simulink model "PV_Array_Code_Gen_PIL"  (R2023b)
settings: Solver=FixedStepAuto  StartTime=0.0  StopTime=86400  FixedStep=1  RelTol=1e-3  EnableMultiTasking=on
libraries: spsSeriesRLCBranchLib x5, spsIdealSwitchLib x3, stm32blockslib x2, spsCurrentMeasurementLib x1, spsDiodeLib x1, spsMosfetLib x1, spsPVArrayLib x1, eePwmGenerator x1, spsVoltageMeasurementLib x1, sps_lib x1
settings Model: STM32="{\"UARTWrite\":{\"ID\":\"PV_Array_Code_Gen:122\"},\"UARTRead\":{\"ID\":\"PV_Array_Code_Gen:121\"}}"  SimulationMode=external  Creator=chate  LastModifiedBy=chate
settings OptimizationCC: EnhancedBackFolding=on  PassReuseOutputArgsAs=Individual arguments  ZeroExternalMemoryAtStartup=off  ZeroInternalMemoryAtStartup=off  MaxStackSize=64  OptimizeBlockOrder=speed  DifferentSizesBufferReuse=on  OptimizationCustomize=off  EfficientTunableParamExpr=on
settings DebuggingCC: AlgebraicLoopMsg=none  ParameterTunabilityLossMsg=error
settings HardwareCC: ProdBitPerPointer=32  ProdBitPerSizeT=32  ProdBitPerPtrDiffT=32  ProdLargestAtomicInteger=Long  ProdLargestAtomicFloat=Double  ProdWordSize=32  ProdLongLongMode=on  ProdHWDeviceType=ARM Compatible->ARM Cortex
settings SFSimCC: MATLABDynamicMemAlloc=off
settings RTWCC: Description=Embedded Coder  SystemTargetFile=ert.tlc  HardwareBoard=STM32F4xx Based  TemplateMakefile=ert_default_tmf  Toolchain=GNU Tools for ARM Embedded Processors  CreateSILPILBlock=PIL
settings CodeAppCC: ForceParamTrailComments=on  IgnoreCustomStorageClasses=off  OperatorAnnotations=on  SimulinkDataObjDesc=on  SFDataObjDesc=on  InsertBlockDesc=on
settings ERTTargetCC: CodeReplacementLibrary=ARM Cortex-M  SupportContinuousTime=on  ExtModeTransport=3  ExtModeStaticAlloc=on  ExtModeStaticAllocSize=2048  ExtModeMexFile=ext_xcp  ExtModeIntrfLevel=Level2 - Open

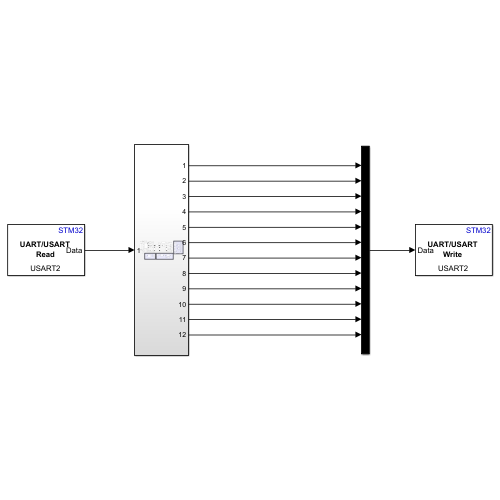
[thumbnail: Simulink's stored preview of the top-level diagram]
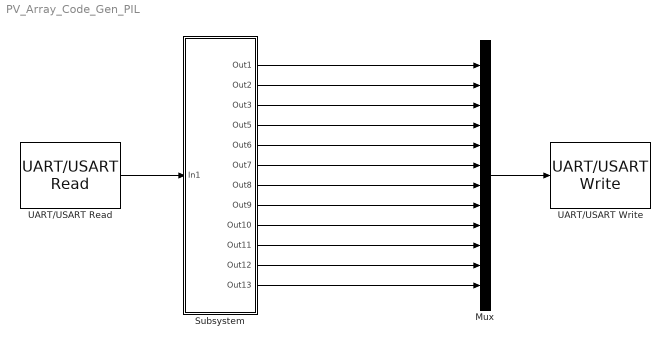
== system PV_Array_Code_Gen_PIL ==
  Mux : Mux  Inputs=12
  Subsystem : Subsystem
  UART/USART Read : stm32blockslib/UART//USART Read  Priority=0  UARTModule=USART2  DataType=double  DataLength=2  BlockingMode=off  BlockingTimeout=0.1  OutputLength=off  OutputStatus=off  SampleTime=1
      settings: LibrarySourceBlock=stm32f4xxblockslib/UART//USART Read
  UART/USART Write : stm32blockslib/UART//USART Write  Priority=1  UARTModule=USART2  LengthOfDataToSend=off  BlockingMode=off  BlockingTimeout=0.1  OutputStatus=off
      settings: LibrarySourceBlock=stm32f4xxblockslib/UART//USART Write
  wires:
  Subsystem/1(Out1) -> Mux/1
  Subsystem/2(Out2) -> Mux/2
  Subsystem/3(Out3) -> Mux/3
  Subsystem/4(Out5) -> Mux/4
  Subsystem/5(Out6) -> Mux/5
  Subsystem/6(Out7) -> Mux/6
  Subsystem/7(Out8) -> Mux/7
  Subsystem/8(Out9) -> Mux/8
  Subsystem/9(Out10) -> Mux/9
  Subsystem/10(Out11) -> Mux/10
  Subsystem/11(Out12) -> Mux/11
  Subsystem/12(Out13) -> Mux/12
  UART/USART Read/1 -> Subsystem/1(In1)
  Mux/1 -> UART/USART Write/1

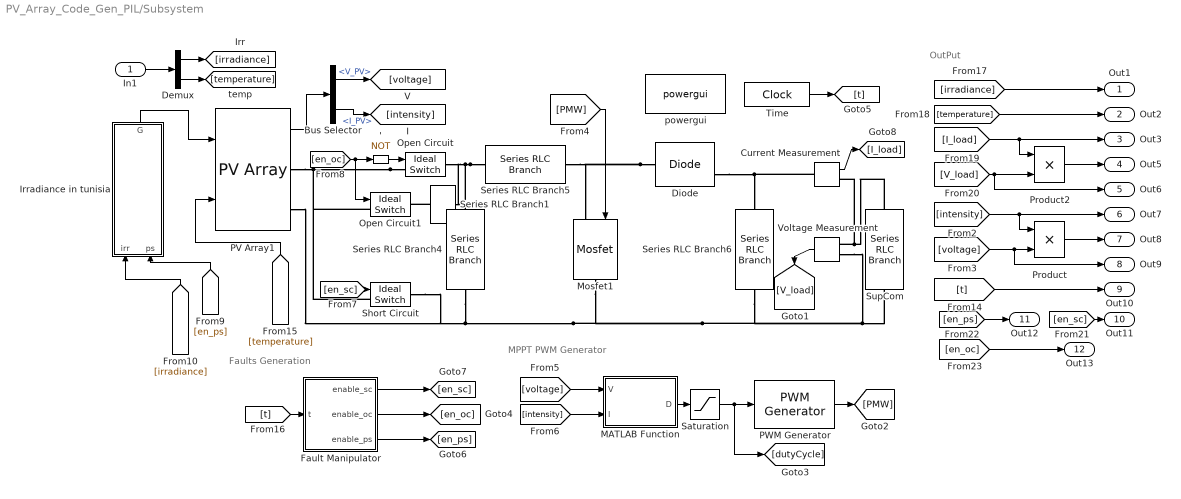
== system PV_Array_Code_Gen_PIL/Subsystem ==
  note: OutPut
  note: Faults Generation
  note: MPPT PWM Generator
  In1 : Inport
  ' : Logic  Operator=NOT  IconShape=distinctive  AllPortsSameDT=off  OutDataTypeStr=boolean
  Bus Selector : BusSelector  OutputSignals=V_PV,I_PV
  Current Measurement : spsCurrentMeasurementLib/Current Measurement  PhasorSimulation=off  OutputType=Complex  PSBequivalent=0
  Demux : Demux  Outputs=2
  Diode : spsDiodeLib/Diode  Ron=0.001  Lon=0  Vf=0.8  IC=0  UseSnubber=0  Rs=100  Cs=1e-7  Measurements=on
  Fault Manipulator : MATLAB Function  TreatAsAtomicUnit=on
  Irradiance in tunisia : MATLAB Function  TreatAsAtomicUnit=on
  MATLAB Function : MATLAB Function  TreatAsAtomicUnit=on
  Mosfet1 : spsMosfetLib/Mosfet  Ron=1e-3  Lon=0  Rd=1e-3  Vfd=0  IC=0  Rs=100  Cs=1e-7  Measurements=off
  Open Circuit : spsIdealSwitchLib/Ideal Switch  Ron=0.000001  Lon=0  IC=1  Rs=0  Cs=0  Measurements=off
  Open Circuit1 : spsIdealSwitchLib/Ideal Switch  Ron=0.000001  Lon=0  IC=0  Rs=0  Cs=0  Measurements=off
  PV Array1 : spsPVArrayLib/PV Array  Npar=3  Nser=15  PlotType=array @ 1000 W/m2 & specified temperatures  S_vec="[ 1000  500  100 ]"  Temp_C_vec="[ 45 25  ]"  ModuleName=User-defined  PlotWhenSelected=off  Pm=451.278  Ncell=60  Voc=49.8  Isc=11.56  Vm=41.1  Im=10.98  beta_Voc_pc=-0.36099  alpha_Isc_pc=0.102  beta_Voc=-0.17977  alpha_Isc=0.011791  IL=11.6189  I0=4.2897e-10  nI=1.3452  Rsh=602.3017  Rs=0.22981  RobustModel=off  RobustCellTemperature=25  BAL=on  Tc=1e-6  Tfilter=5e-5
  PWM Generator : eePwmGenerator/PWM Generator  CarrCount=Up  Tper=10  Tdelay=0  Ts=1
  Product : Product
  Product2 : Product
  Saturation : Saturate  UpperLimit=1  LowerLimit=0
  Series RLC Branch1 : spsSeriesRLCBranchLib/Series RLC Branch  LConnTagsString=__new0  RConnTagsString=__new0  BranchType=R  Resistance=7.3  Inductance=1.63e-2  SetiL0=off  InitialCurrent=0  Capacitance=1e-3  Setx0=off  InitialVoltage=0  Measurements=None
  Series RLC Branch4 : spsSeriesRLCBranchLib/Series RLC Branch  LConnTagsString=__new0  RConnTagsString=__new0  BranchType=C  Resistance=1  Inductance=1e-3  SetiL0=off  InitialCurrent=0  Capacitance=46.6e-2  Setx0=off  InitialVoltage=0  Measurements=None
  Series RLC Branch5 : spsSeriesRLCBranchLib/Series RLC Branch  LConnTagsString=__new0  RConnTagsString=__new0  BranchType=L  Resistance=1  Inductance=1.63e-2  SetiL0=off  InitialCurrent=0  Capacitance=1e-3  Setx0=off  InitialVoltage=0  Measurements=None
  Series RLC Branch6 : spsSeriesRLCBranchLib/Series RLC Branch  LConnTagsString=__new0  RConnTagsString=__new0  BranchType=C  Resistance=1  Inductance=1e-3  SetiL0=off  InitialCurrent=0  Capacitance=63e-2  Setx0=off  InitialVoltage=0  Measurements=None
  Short Circuit : spsIdealSwitchLib/Ideal Switch  Ron=0.000001  Lon=0  IC=0  Rs=0  Cs=0  Measurements=off
  SupCom : spsSeriesRLCBranchLib/Series RLC Branch  LConnTagsString=__new0  RConnTagsString=__new0  BranchType=R  Resistance=18.5  Inductance=1e-3  SetiL0=off  InitialCurrent=0  Capacitance=1e-3  Setx0=off  InitialVoltage=0  Measurements=None
  Time : DigitalClock
  Voltage Measurement : spsVoltageMeasurementLib/Voltage Measurement  PhasorSimulation=off  OutputType=Complex  PSBequivalent=0
  powergui : sps_lib/powergui  Priority=1  SimulationMode=Discrete  SampleTime=1  frequency=60  Iterations=50  frequencyindice=0  Pbase=100e6  ErrMax=1e-4  UnitsV=kV  UnitsW=MW  buscounter=0  FunctionMessages=off  echomessages=off  EnableUseOfTLC=off  CurrentSourceSwitches=off  DisableSnubberDevices=off  DisableRonSwitches=off  DisableVfSwitches=off  DisplayEquations=off  AutomaticDiscreteSolvers=off  SolverType=Tustin/Backward Euler (TBE)  Interpol=off  ExternalGateDelay=off  methode=off  Ts=100  x0status=blocks  SPID=on  SwTol=0  HookPort=off  NonlinearTolerance=1e-4  nMaxIteration=100  ContinueOnMaxIteration=off  RestoreLinks=warning  ResistiveCurrentMeasurement=off  Frange=[0:2:500]  Ylog=off  Xlog=on  ShowGrid=off  save=off  variable=ZData  structure=0  ZoomFFT=off  StartTime=0.0  cycles=1  DisplayStyle=1  fundamental=60  FreqAxis=off  MaxFrequency=1000  frequencyindicesteady=1  RmsSteady=1  display=off
  Out1 : Outport
  Out2 : Outport  Port=2
  Out3 : Outport  Port=3
  Out5 : Outport  Port=4
  Out6 : Outport  Port=5
  Out7 : Outport  Port=6
  Out8 : Outport  Port=7
  Out9 : Outport  Port=8
  Out10 : Outport  Port=9
  Out11 : Outport  Port=10
  Out12 : Outport  Port=11
  Out13 : Outport  Port=12
  wires:
  [temperature] -> PV Array1/2
  [en_oc] -> '/1, Open Circuit1/1
  [intensity] -> MATLAB Function/2(I)
  [en_oc] -> Out13/1
  Fault Manipulator/3(enable_ps) -> [en_ps]
  Bus Selector/2 -> [intensity]  "<I_PV>"
  Fault Manipulator/2(enable_oc) -> [en_oc]
  Irradiance in tunisia/1(G) -> PV Array1/1
  [V_load] -> Out6/1, Product2/2
  Current Measurement/1 -> [I_load]
  [temperature] -> Out2/1
  Product/1 -> Out8/1
  Demux/1 -> [irradiance]
  [voltage] -> MATLAB Function/1(V)
  [I_load] -> Out3/1, Product2/1
  Voltage Measurement/1 -> [V_load]
  PWM Generator/1 -> [PMW]
  [PMW] -> Mosfet1/1
  MATLAB Function/1(D) -> Saturation/1
  Fault Manipulator/1(enable_sc) -> [en_sc]
  [voltage] -> Out9/1, Product/2
  [en_ps] -> Irradiance in tunisia/2(ps)
  PV Array1/1 -> Bus Selector/1
  [intensity] -> Out7/1, Product/1
  Bus Selector/1 -> [voltage]  "<V_PV>"
  Time/1 -> [t]
  [t] -> Fault Manipulator/1(t)
  [irradiance] -> Irradiance in tunisia/1(irr)
  Demux/2 -> [temperature]
  Saturation/1 -> PWM Generator/1, [dutyCycle]
  '/1 -> Open Circuit/1
  [en_sc] -> Out11/1
  [irradiance] -> Out1/1
  [en_sc] -> Short Circuit/1
  Product2/1 -> Out5/1
  In1/1 -> Demux/1
  [t] -> Out10/1
  [en_ps] -> Out12/1
  connections:
  Series RLC Branch5/LConn1 -- Series RLC Branch4/LConn1 -- Series RLC Branch1/RConn1 -- Open Circuit/RConn1
  Diode/RConn1 -- Current Measurement/LConn1 -- Series RLC Branch6/LConn1
  Open Circuit/LConn1 -- PV Array1/RConn1 -- Open Circuit1/LConn1 -- Short Circuit/LConn1
  Voltage Measurement/LConn1 -- SupCom/LConn1 -- Current Measurement/RConn1
  Diode/LConn1 -- Series RLC Branch5/RConn1 -- Mosfet1/LConn1
  Voltage Measurement/LConn2 -- Series RLC Branch6/RConn1 -- Mosfet1/RConn1 -- Series RLC Branch4/RConn1 -- Short Circuit/RConn1 -- PV Array1/RConn2 -- SupCom/RConn1
  Series RLC Branch1/LConn1 -- Open Circuit1/RConn1

== matlab function PV_Array_Code_Gen_PIL/Subsystem/Irradiance in tunisia ==
  data: irr input; G output; ps input
function G = irradiance_profile_tunisia(irr, ps)
    
    G = max(0, irr);

    if ps == 1
        G = 0.85 * G;  % Reduce irradiance to 85%
    end
end

== matlab function PV_Array_Code_Gen_PIL/Subsystem/Fault Manipulator ==
  data: t input; enable_sc output; enable_oc output; enable_ps output
function [enable_sc, enable_oc, enable_ps] = faults(t)
    % Time-dependent fault trigger system
    % Fault probability per second
    persistent fault_type fault_start_time fault_duration

    % Parameters
    fault_probability = 0.05;  % chance of a fault occurring at each call
    enable_sc = 0;
    enable_oc = 0;
    enable_ps = 0;

    % First call init
    if isempty(fault_type)
        fault_type = 0;
        fault_duration = 0;
        fault_start_time = -Inf;
    end

    % Check if current fault is active
    if t < fault_start_time + fault_duration
        % Maintain the current fault
        switch fault_type
            case 1
                enable_sc = 1;
                enable_oc = 0;
                enable_ps = 0;
            case 2
                enable_sc = 0;
                enable_oc = 1;
                enable_ps = 0;
            case 3
                enable_sc = 0;
                enable_oc = 0;
                enable_ps = 1;
        end
    else
        % No active fault, decide if a new one should start
        if rand < fault_probability
            fault_duration = randi(50) + 10;
            fault_type = randi(3);  % random fault (1=SC, 2=OC, 3=PS)
            fault_start_time = t;
        else
            % No fault
            fault_type = 0;
            enable_sc = 0;
            enable_oc = 0;
            enable_ps = 0;
        end
    end
end

== matlab function PV_Array_Code_Gen_PIL/Subsystem/MATLAB Function ==
  data: V input; D output; I input
function D = MPPT(V, I)
    persistent Vold Pold Dold;

    % MPPT parameters
    deltaD = 0.005;    % Step size
    P = V * I;
    
    % Initialize with better startup conditions
    if isempty(Vold)
        Vold = V;
        Pold = P;
        Dold = 0.175;  % Starting duty cycle
    end
    
    % Startup protection
    if V < 10  % If voltage is too low
        D = 0.05;  % Minimum duty cycle to build up voltage
        
        % Update persistent variables
        Vold = V;
        Pold = P;
        Dold = D;
        return;
    end
    
    % Modified P&O algorithm with additional checks
    if abs(V - Vold) < 0.1  % If voltage barely changed
        deltaD = 0.01;  % Increase step size
    end

    if (P - Pold) ~= 0
        if (P - Pold) > 0
            if (V - Vold) > 0
                D = Dold + deltaD;
            else
                D = Dold - deltaD;
            end
        else
            if (V - Vold) > 0
                D = Dold - deltaD;
            else
                D = Dold + deltaD;
            end
        end
    else
        D = Dold;
    end
    
    % Update old values
    Vold = V;
    Pold = P;
    Dold = D;
    D = max(min(D, 2000), 0.05);
end
